simulink model "three_phase_solar_grid"  (R2020b)
settings: Solver=VariableStepAuto  StartTime=0.0  StopTime=0.8  RelTol=1e-6
libraries: powerlib x26, powerlib_meascontrol x3, simulink x3, re_lib x1
settings Model: Creator=a6039  LastModifiedBy=a6039

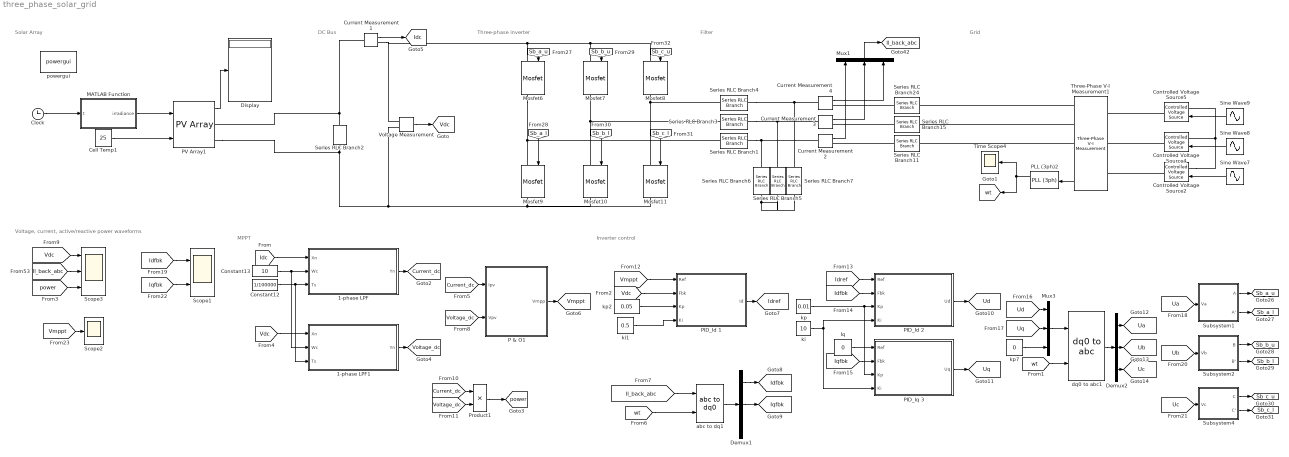
== system three_phase_solar_grid ==
  note: Filter
  note: Solar Array
  note: MPPT
  note: Three-phase inverter
  note: Inverter control
  note: Voltage, current, active/reactive power waveforms
  note: DC Bus
  note: Grid
  1-phase LPF : Subsystem  TreatAsAtomicUnit=on
  1-phase LPF1 : Subsystem  TreatAsAtomicUnit=on
  Cell Temp1 : Constant  Value=25
  Clock : Clock
  Constant12 : Constant  Value=1/100000
  Constant13 : Constant  Value=10
  Controlled Voltage Source2 : powerlib/Electrical Sources/Controlled Voltage Source  Initialize=on  Source_Type=AC  Amplitude=0  Phase=0  Frequency=0  Measurements=None
  Controlled Voltage Source4 : powerlib/Electrical Sources/Controlled Voltage Source  Initialize=on  Source_Type=AC  Amplitude=0  Phase=0  Frequency=0  Measurements=None
  Controlled Voltage Source5 : powerlib/Electrical Sources/Controlled Voltage Source  Initialize=on  Source_Type=AC  Amplitude=0  Phase=0  Frequency=0  Measurements=None
  Current Measurement{1..4} (4 alike) : powerlib/Measurements/Current Measurement  PhasorSimulation=off  OutputType=Complex  PSBequivalent=0
  Demux1 : Demux  Outputs=3
  Demux2 : Demux  Outputs=3
  Display : Display
      settings: Decimation=5
  Iq : Constant  Value=0
  MATLAB Function : MATLAB Function  TreatAsAtomicUnit=on
  Mosfet{6..11} (6 alike) : powerlib/Power Electronics/Mosfet  Ron=0.1  Lon=0  Rd=0.01  Vfd=0  IC=0  Rs=1e5  Cs=inf  Measurements=on
  Mux1 : Mux  Inputs=3
  Mux3 : Mux  Inputs=3
  P & O1 : Subsystem
  PID_Id 1 : Subsystem
  PID_Id 2 : Subsystem
  PID_Iq 3 : Subsystem
  PLL (3ph)2 : powerlib_meascontrol/PLL/PLL (3ph)  Fmin=45  Par_Init=[0, 60]  ParK=[180, 3200, 1]  TcD=1e-4  MaxRateChangeFreq=12  FilterCutOffFreq=25  Ts=0  AGC=on
  PV Array1 : re_lib/Solar/PV Array  Npar=40  Nser=10  PlotType=array @ 1000 W/m2 & specified temperatures  S_vec="[ 1000  800  600 400 200 ]"  Temp_C_vec="[ 45 25  ]"  ModuleName=Ablytek 5MN6C175-A0  PlotWhenSelected=off  Pm=175.0914  Ncell=72  Voc=43.99  Isc=5.17  Vm=36.63  Im=4.78  beta_Voc_pc=-0.3616  alpha_Isc_pc=0.041509  beta_Voc=-0.15907  alpha_Isc=0.002146  IL=5.178  I0=1.7842e-10  nI=0.98852  Rsh=249.6758  Rs=0.38412  RobustModel=off  RobustCellTemperature=313.3991  BAL=off  Tc=1e-6  Tfilter=5e-4
  Product1 : Product
  Scope1 : Scope  NumInputPorts=2
  Scope2 : Scope
  Scope3 : Scope  NumInputPorts=3
  Series RLC Branch1 : powerlib/Elements/Series RLC Branch  LConnTagsString=__new0  RConnTagsString=__new0  BranchType=L  Resistance=1  Inductance=1e-3  SetiL0=off  InitialCurrent=0  Capacitance=1e-3  Setx0=off  InitialVoltage=0  Measurements=None
  Series RLC Branch11 : powerlib/Elements/Series RLC Branch  LConnTagsString=__new0  RConnTagsString=__new0  BranchType=RL  Resistance=0.1  Inductance=1e-9  SetiL0=off  InitialCurrent=0  Capacitance=1e-6  Setx0=off  InitialVoltage=0  Measurements=None
  Series RLC Branch15 : powerlib/Elements/Series RLC Branch  LConnTagsString=__new0  RConnTagsString=__new0  BranchType=RL  Resistance=0.1  Inductance=1e-9  SetiL0=off  InitialCurrent=0  Capacitance=1e-6  Setx0=off  InitialVoltage=0  Measurements=None
  Series RLC Branch2 : powerlib/Elements/Series RLC Branch  LConnTagsString=__new0  RConnTagsString=__new0  BranchType=RC  Resistance=1e-8  Inductance=250e-6  SetiL0=off  InitialCurrent=0  Capacitance=1e-3  Setx0=off  InitialVoltage=300  Measurements=None
  Series RLC Branch24 : powerlib/Elements/Series RLC Branch  LConnTagsString=__new0  RConnTagsString=__new0  BranchType=RL  Resistance=0.1  Inductance=1e-9  SetiL0=off  InitialCurrent=0  Capacitance=1e-6  Setx0=off  InitialVoltage=0  Measurements=None
  Series RLC Branch3 : powerlib/Elements/Series RLC Branch  LConnTagsString=__new0  RConnTagsString=__new0  BranchType=L  Resistance=1  Inductance=1e-3  SetiL0=off  InitialCurrent=0  Capacitance=1e-3  Setx0=off  InitialVoltage=0  Measurements=None
  Series RLC Branch4 : powerlib/Elements/Series RLC Branch  LConnTagsString=__new0  RConnTagsString=__new0  BranchType=L  Resistance=1  Inductance=1e-3  SetiL0=off  InitialCurrent=0  Capacitance=1e-3  Setx0=off  InitialVoltage=0  Measurements=None
  Series RLC Branch5 : powerlib/Elements/Series RLC Branch  LConnTagsString=__new0  RConnTagsString=__new0  BranchType=C  Resistance=1  Inductance=10e-4  SetiL0=off  InitialCurrent=0  Capacitance=1e-4  Setx0=off  InitialVoltage=0  Measurements=None
  Series RLC Branch6 : powerlib/Elements/Series RLC Branch  LConnTagsString=__new0  RConnTagsString=__new0  BranchType=C  Resistance=1  Inductance=10e-4  SetiL0=off  InitialCurrent=0  Capacitance=1e-4  Setx0=off  InitialVoltage=0  Measurements=None
  Series RLC Branch7 : powerlib/Elements/Series RLC Branch  LConnTagsString=__new0  RConnTagsString=__new0  BranchType=C  Resistance=1  Inductance=10e-4  SetiL0=off  InitialCurrent=0  Capacitance=1e-4  Setx0=off  InitialVoltage=0  Measurements=None
  Sine Wave7 : Sin  Amplitude=169.7  Frequency=60*2*pi  SampleTime=0
  Sine Wave8 : Sin  Amplitude=169.7  Frequency=60*2*pi  Phase=-2*pi/3  SampleTime=0
  Sine Wave9 : Sin  Amplitude=169.7  Frequency=60*2*pi  Phase=-4*pi/3  SampleTime=0
  Subsystem1 : Subsystem
  Subsystem2 : Subsystem
  Subsystem4 : Subsystem
  Three-Phase V-I Measurement1 : powerlib/Measurements/Three-Phase V-I Measurement  VoltageMeasurement=phase-to-phase  SetLabelV=off  LabelV=Vabc  Vpu=off  VpuLL=off  CurrentMeasurement=yes  SetLabelI=off  LabelI=Iabc  Ipu=off  Pbase=100e6  Vbase=500e3  OutputType=Complex  PhasorSimulation=off  PSBequivalent=0
  Time Scope4 : Scope
  Voltage Measurement : powerlib/Measurements/Voltage Measurement  PhasorSimulation=off  OutputType=Complex  PSBequivalent=0
  abc to dq1 : powerlib_meascontrol/Transformations/abc to dq0  Alignment=Aligned with phase A axis
  dq0 to abc1 : powerlib_meascontrol/Transformations/dq0 to abc  Alignment=Aligned with phase A axis
  ki : Constant  Value=10
  ki1 : Constant  Value=0.5
  kp : Constant  Value=0.01
  kp2 : Constant  Value=0.05
  kp7 : Constant  Value=0
  powergui : powerlib/powergui  Priority=1  SimulationMode=Discrete  SampleTime=1e-7  frequency=60  Iterations=50  frequencyindice=0  Pbase=100e6  ErrMax=1e-4  UnitsV=kV  UnitsW=MW  buscounter=0  FunctionMessages=off  echomessages=off  EnableUseOfTLC=off  CurrentSourceSwitches=off  DisableSnubberDevices=off  DisableRonSwitches=off  DisableVfSwitches=off  DisplayEquations=off  AutomaticDiscreteSolvers=off  SolverType=Tustin/Backward Euler (TBE)  Interpol=off  ExternalGateDelay=off  methode=off  Ts=100  x0status=blocks  SPID=on  SwTol=0  HookPort=off  NonlinearTolerance=1e-4  nMaxIteration=100  ContinueOnMaxIteration=off  RestoreLinks=warning  ResistiveCurrentMeasurement=off  Frange=[0:2:500]  Ylog=off  Xlog=on  ShowGrid=off  save=off  variable=ZData  structure=current  ZoomFFT=off  StartTime=0.2  cycles=20  DisplayStyle=1  fundamental=50  FreqAxis=off  MaxFrequency=500  frequencyindicesteady=1  RmsSteady=1  display=off
  tag scope: Current_dc=global, Idc=global, Idfbk=global, Idref=global, Il_back_abc=global, Iqfbk=global, Sb_a_l=global, Sb_a_u=global, Sb_b_l=global, Sb_b_u=global, Sb_c_l=global, Sb_c_u=global, Ua=global, Ub=global, Uc=global, Ud=global, Uq=global, Vdc=global, Vmppt=global, Voltage_dc=global, power=global, wt=global
  wires:
  Current Measurement2/1 -> Mux1/1
  Current Measurement3/1 -> Mux1/2
  Current Measurement4/1 -> Mux1/3
  [Il_back_abc] -> Scope3/2
  Iq/1 -> PID_Iq 3/1(Ref)
  abc to dq1/1 -> Demux1/1
  [wt] -> dq0 to abc1/2
  kp/1 -> PID_Iq 3/3(Kp), PID_Id 2/3(Kp)
  ki/1 -> PID_Id 2/4(Ki), PID_Iq 3/4(Ki)
  Mux3/1 -> dq0 to abc1/1
  [wt] -> abc to dq1/2
  dq0 to abc1/1 -> Demux2/1
  PLL (3ph)2/2 -> [wt], Time Scope4/1
  Sine Wave8/1 -> Controlled Voltage Source4/1
  Sine Wave9/1 -> Controlled Voltage Source5/1
  Sine Wave7/1 -> Controlled Voltage Source2/1
  Three-Phase V-I Measurement1/1 -> PLL (3ph)2/1
  [Il_back_abc] -> abc to dq1/1
  Mux1/1 -> [Il_back_abc]
  Cell Temp1/1 -> PV Array1/2
  [Sb_a_u] -> Mosfet6/1
  [Sb_b_u] -> Mosfet7/1
  [Sb_c_u] -> Mosfet8/1
  [Sb_a_l] -> Mosfet9/1
  [Sb_b_l] -> Mosfet10/1
  [Sb_c_l] -> Mosfet11/1
  Voltage Measurement/1 -> [Vdc]
  PV Array1/1 -> Display/1
  [Vdc] -> PID_Id 1/2(Fbk)
  kp2/1 -> PID_Id 1/3(Kp)
  ki1/1 -> PID_Id 1/4(Ki)
  Constant12/1 -> 1-phase LPF1/3(Ts), 1-phase LPF/3(Ts)
  Constant13/1 -> 1-phase LPF1/2(Wc), 1-phase LPF/2(Wc)
  [Idc] -> 1-phase LPF/1(Xn)
  [Vdc] -> 1-phase LPF1/1(Xn)
  Subsystem1/1(A) -> [Sb_a_u]
  Subsystem1/2(A') -> [Sb_a_l]
  Subsystem2/1(B) -> [Sb_b_u]
  Subsystem2/2(B') -> [Sb_b_l]
  Subsystem4/1(C) -> [Sb_c_u]
  Subsystem4/2(C') -> [Sb_c_l]
  kp7/1 -> Mux3/3
  [Vdc] -> Scope3/1
  [power] -> Scope3/3
  Product1/1 -> [power]
  MATLAB Function/1(irradiance) -> PV Array1/1
  Clock/1 -> MATLAB Function/1(t)
  Current Measurement1/1 -> [Idc]
  1-phase LPF/1(Yn) -> [Current_dc]
  1-phase LPF1/1(Yn) -> [Voltage_dc]
  [Current_dc] -> P & O1/1(Ipv)
  [Voltage_dc] -> P & O1/2(Vpv)
  [Current_dc] -> Product1/1
  [Voltage_dc] -> Product1/2
  P & O1/1(Vmpp) -> [Vmppt]
  [Vmppt] -> PID_Id 1/1(Ref)
  PID_Id 1/1(Id) -> [Idref]
  [Idref] -> PID_Id 2/1(Ref)
  Demux1/1 -> [Idfbk]
  Demux1/2 -> [Iqfbk]
  [Idfbk] -> PID_Id 2/2(Fbk)
  [Iqfbk] -> PID_Iq 3/2(Fbk)
  PID_Id 2/1(Ud) -> [Ud]
  PID_Iq 3/1(Uq) -> [Uq]
  [Ud] -> Mux3/1
  [Uq] -> Mux3/2
  Demux2/1 -> [Ua]
  Demux2/2 -> [Ub]
  Demux2/3 -> [Uc]
  [Ua] -> Subsystem1/1(Va)
  [Ub] -> Subsystem2/1(Vb)
  [Uc] -> Subsystem4/1(Vc)
  [Idfbk] -> Scope1/1
  [Iqfbk] -> Scope1/2
  [Vmppt] -> Scope2/1
  connections:
  Mosfet6/LConn1 -- Voltage Measurement/LConn1 -- Current Measurement1/RConn1 -- Mosfet8/LConn1 -- Mosfet7/LConn1
  Mosfet11/LConn1 -- Series RLC Branch4/LConn1 -- Mosfet8/RConn1
  Mosfet10/LConn1 -- Series RLC Branch3/LConn1 -- Mosfet7/RConn1
  Mosfet6/RConn1 -- Mosfet9/LConn1 -- Series RLC Branch1/LConn1
  Controlled Voltage Source2/LConn1 -- Controlled Voltage Source5/LConn1 -- Controlled Voltage Source4/LConn1
  Controlled Voltage Source5/RConn1 -- Three-Phase V-I Measurement1/LConn3
  Controlled Voltage Source2/RConn1 -- Three-Phase V-I Measurement1/LConn1
  Controlled Voltage Source4/RConn1 -- Three-Phase V-I Measurement1/LConn2
  Series RLC Branch2/LConn1 -- PV Array1/RConn2 -- Voltage Measurement/LConn2 -- Mosfet11/RConn1 -- Mosfet10/RConn1 -- Mosfet9/RConn1
  Series RLC Branch6/RConn1 -- Series RLC Branch7/RConn1 -- Series RLC Branch5/RConn1
  Three-Phase V-I Measurement1/RConn1 -- Series RLC Branch11/RConn1
  Three-Phase V-I Measurement1/RConn2 -- Series RLC Branch15/RConn1
  Three-Phase V-I Measurement1/RConn3 -- Series RLC Branch24/RConn1
  Series RLC Branch1/RConn1 -- Series RLC Branch6/LConn1 -- Current Measurement2/LConn1
  Series RLC Branch3/RConn1 -- Series RLC Branch5/LConn1 -- Current Measurement3/LConn1
  Series RLC Branch4/RConn1 -- Series RLC Branch7/LConn1 -- Current Measurement4/LConn1
  Series RLC Branch24/LConn1 -- Current Measurement4/RConn1
  Series RLC Branch15/LConn1 -- Current Measurement3/RConn1
  Series RLC Branch11/LConn1 -- Current Measurement2/RConn1
  Series RLC Branch2/RConn1 -- PV Array1/RConn1 -- Current Measurement1/LConn1

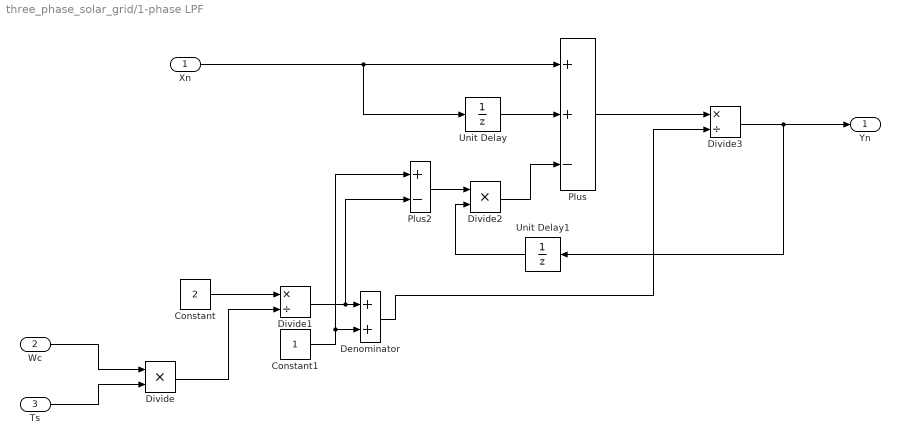
== system three_phase_solar_grid/1-phase LPF ==
  Xn : Inport
  Wc : Inport  Port=2
  Ts : Inport  Port=3
  Constant : Constant  Value=2
  Constant1 : Constant
  Denominator : Sum
  Divide : Product  Inputs=**
  Divide1 : Product  Inputs=*/
  Divide2 : Product  Inputs=**
  Divide3 : Product  Inputs=*/
  Plus : Sum  Inputs=++-
  Plus2 : Sum  Inputs=+-
  Unit Delay : UnitDelay  SampleTime=-1  HasFrameUpgradeWarning=on
  Unit Delay1 : UnitDelay  SampleTime=-1  HasFrameUpgradeWarning=on
  Yn : Outport
  wires:
  Xn/1 -> Unit Delay/1, Plus/1
  Unit Delay/1 -> Plus/2
  Wc/1 -> Divide/1
  Ts/1 -> Divide/2
  Divide/1 -> Divide1/2
  Constant/1 -> Divide1/1
  Divide1/1 -> Plus2/2, Denominator/1
  Constant1/1 -> Plus2/1, Denominator/2
  Plus2/1 -> Divide2/1
  Unit Delay1/1 -> Divide2/2
  Plus/1 -> Divide3/1
  Denominator/1 -> Divide3/2
  Divide3/1 -> Unit Delay1/1, Yn/1
  Divide2/1 -> Plus/3

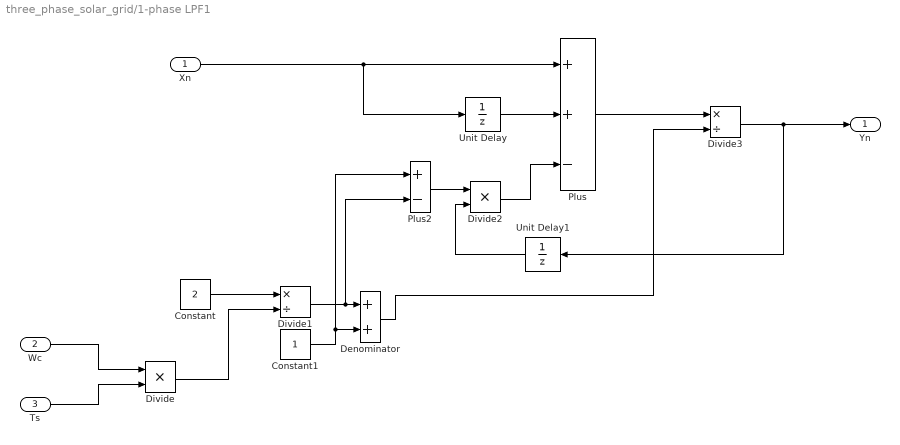
== system three_phase_solar_grid/1-phase LPF1 ==
  Xn : Inport
  Wc : Inport  Port=2
  Ts : Inport  Port=3
  Constant : Constant  Value=2
  Constant1 : Constant
  Denominator : Sum
  Divide : Product  Inputs=**
  Divide1 : Product  Inputs=*/
  Divide2 : Product  Inputs=**
  Divide3 : Product  Inputs=*/
  Plus : Sum  Inputs=++-
  Plus2 : Sum  Inputs=+-
  Unit Delay : UnitDelay  SampleTime=-1  HasFrameUpgradeWarning=on
  Unit Delay1 : UnitDelay  SampleTime=-1  HasFrameUpgradeWarning=on
  Yn : Outport
  wires:
  Xn/1 -> Unit Delay/1, Plus/1
  Unit Delay/1 -> Plus/2
  Wc/1 -> Divide/1
  Ts/1 -> Divide/2
  Divide/1 -> Divide1/2
  Constant/1 -> Divide1/1
  Divide1/1 -> Plus2/2, Denominator/1
  Constant1/1 -> Plus2/1, Denominator/2
  Plus2/1 -> Divide2/1
  Unit Delay1/1 -> Divide2/2
  Plus/1 -> Divide3/1
  Denominator/1 -> Divide3/2
  Divide3/1 -> Unit Delay1/1, Yn/1
  Divide2/1 -> Plus/3

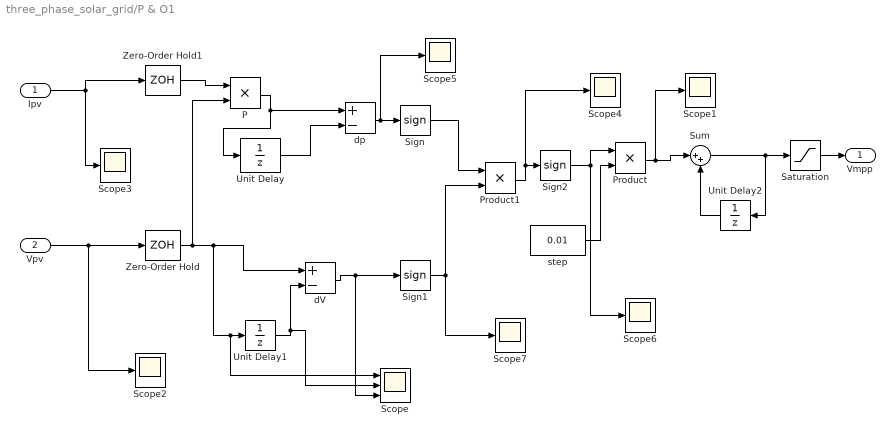
== system three_phase_solar_grid/P & O1 ==
  Ipv : Inport
  Vpv : Inport  Port=2
  P : Product  RndMeth=Zero
  Product : Product  RndMeth=Zero
  Product1 : Product  RndMeth=Zero
  Saturation : Saturate  UpperLimit=450  LowerLimit=0  LinearizeAsGain=off  ZeroCross=off
  Scope : Scope  NumInputPorts=3
  Scope{1..7} (7 alike) : Scope
  Sign : Signum
  Sign1 : Signum
  Sign2 : Signum
  Sum : Sum  Inputs=|++
  Unit Delay : UnitDelay  SampleTime=-1  HasFrameUpgradeWarning=on
  Unit Delay1 : UnitDelay  SampleTime=-1  HasFrameUpgradeWarning=on
  Unit Delay2 : UnitDelay  InitialCondition=400  SampleTime=-1  HasFrameUpgradeWarning=on
  Zero-Order Hold : ZeroOrderHold  SampleTime=1/100000
  Zero-Order Hold1 : ZeroOrderHold  SampleTime=1/100000
  dV : Sum  Inputs=+-
  dp : Sum  Inputs=+-
  step : Constant  Value=0.01
  Vmpp : Outport
  wires:
  Unit Delay1/1 -> dV/2, Scope/2
  Unit Delay/1 -> dp/2
  dV/1 -> Sign1/1, Scope/3
  step/1 -> Product/2
  Product/1 -> Sum/1, Scope1/1
  Sign/1 -> Product1/1
  Sign1/1 -> Product1/2, Scope7/1
  Product1/1 -> Sign2/1, Scope4/1
  Ipv/1 -> Scope3/1, Zero-Order Hold1/1
  Vpv/1 -> Zero-Order Hold/1, Scope2/1
  P/1 -> Unit Delay/1, dp/1
  dp/1 -> Sign/1, Scope5/1
  Sign2/1 -> Product/1, Scope6/1
  Sum/1 -> Saturation/1, Unit Delay2/1
  Unit Delay2/1 -> Sum/2
  Zero-Order Hold/1 -> P/2, Scope/1, Unit Delay1/1, dV/1
  Zero-Order Hold1/1 -> P/1
  Saturation/1 -> Vmpp/1

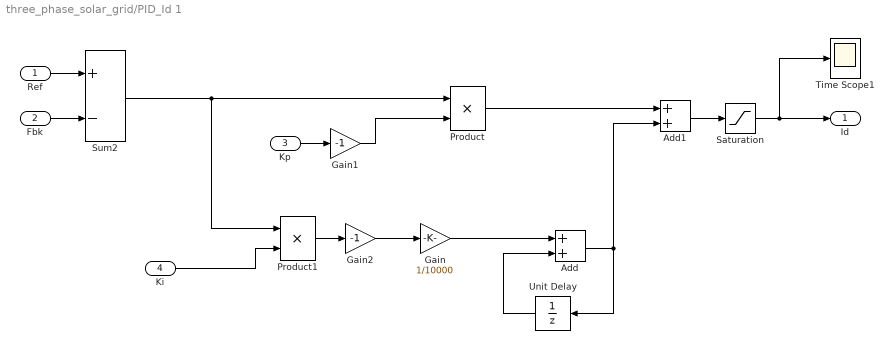
== system three_phase_solar_grid/PID_Id 1 ==
  Ref : Inport
  Fbk : Inport  Port=2
  Kp : Inport  Port=3
  Ki : Inport  Port=4
  Add : Sum
  Add1 : Sum
  Gain : Gain  Gain=1/10000
  Gain1 : Gain  Gain=-1
  Gain2 : Gain  Gain=-1
  Product : Product  OutDataTypeStr=Inherit: Same as first input
  Product1 : Product  OutDataTypeStr=Inherit: Same as first input
  Saturation : Saturate  UpperLimit=1000  LowerLimit=0  LinearizeAsGain=off  ZeroCross=off
  Sum2 : Sum  Inputs=+-
  Time Scope1 : Scope
  Unit Delay : UnitDelay  SampleTime=-1  HasFrameUpgradeWarning=on
  Id : Outport
  wires:
  Sum2/1 -> Product1/1, Product/1
  Fbk/1 -> Sum2/2
  Ref/1 -> Sum2/1
  Product1/1 -> Gain2/1
  Add/1 -> Unit Delay/1, Add1/2
  Product/1 -> Add1/1
  Gain/1 -> Add/1
  Unit Delay/1 -> Add/2
  Kp/1 -> Gain1/1
  Ki/1 -> Product1/2
  Gain1/1 -> Product/2
  Gain2/1 -> Gain/1
  Add1/1 -> Saturation/1
  Saturation/1 -> Time Scope1/1, Id/1

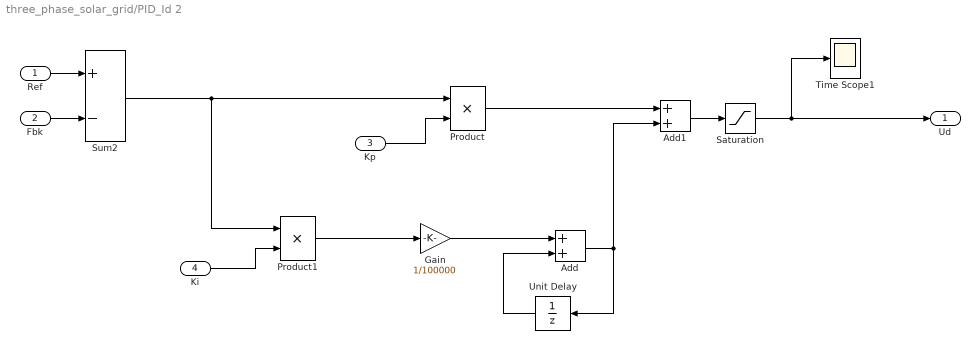
== system three_phase_solar_grid/PID_Id 2 ==
  Ref : Inport
  Fbk : Inport  Port=2
  Kp : Inport  Port=3
  Ki : Inport  Port=4
  Add : Sum
  Add1 : Sum
  Gain : Gain  Gain=1/100000
  Product : Product  OutDataTypeStr=Inherit: Same as first input
  Product1 : Product  OutDataTypeStr=Inherit: Same as first input
  Saturation : Saturate  UpperLimit=500  LowerLimit=-500  LinearizeAsGain=off  ZeroCross=off
  Sum2 : Sum  Inputs=+-
  Time Scope1 : Scope
  Unit Delay : UnitDelay  InitialCondition=400  SampleTime=-1  HasFrameUpgradeWarning=on
  Ud : Outport
  wires:
  Add1/1 -> Saturation/1
  Sum2/1 -> Product1/1, Product/1
  Fbk/1 -> Sum2/2
  Ref/1 -> Sum2/1
  Kp/1 -> Product/2
  Ki/1 -> Product1/2
  Product1/1 -> Gain/1
  Add/1 -> Unit Delay/1, Add1/2
  Product/1 -> Add1/1
  Saturation/1 -> Time Scope1/1, Ud/1
  Gain/1 -> Add/1
  Unit Delay/1 -> Add/2

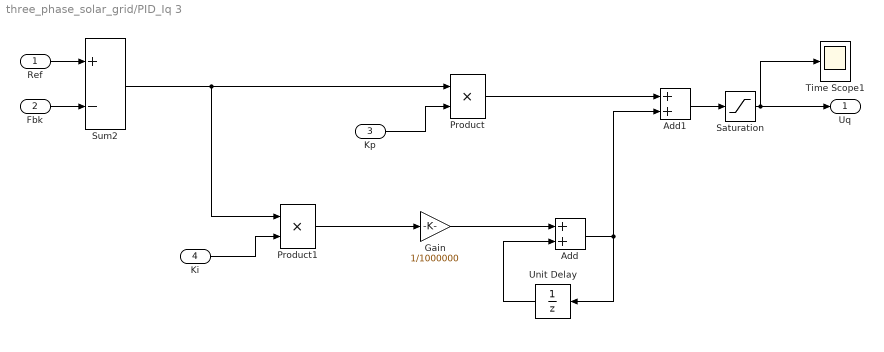
== system three_phase_solar_grid/PID_Iq 3 ==
  Ref : Inport
  Fbk : Inport  Port=2
  Kp : Inport  Port=3
  Ki : Inport  Port=4
  Add : Sum
  Add1 : Sum
  Gain : Gain  Gain=1/1000000
  Product : Product  OutDataTypeStr=Inherit: Same as first input
  Product1 : Product  OutDataTypeStr=Inherit: Same as first input
  Saturation : Saturate  UpperLimit=500  LowerLimit=-500  LinearizeAsGain=off  ZeroCross=off
  Sum2 : Sum  Inputs=+-
  Time Scope1 : Scope
  Unit Delay : UnitDelay  SampleTime=-1  HasFrameUpgradeWarning=on
  Uq : Outport
  wires:
  Add1/1 -> Saturation/1
  Sum2/1 -> Product1/1, Product/1
  Fbk/1 -> Sum2/2
  Ref/1 -> Sum2/1
  Kp/1 -> Product/2
  Ki/1 -> Product1/2
  Product1/1 -> Gain/1
  Add/1 -> Unit Delay/1, Add1/2
  Product/1 -> Add1/1
  Gain/1 -> Add/1
  Unit Delay/1 -> Add/2
  Saturation/1 -> Time Scope1/1, Uq/1

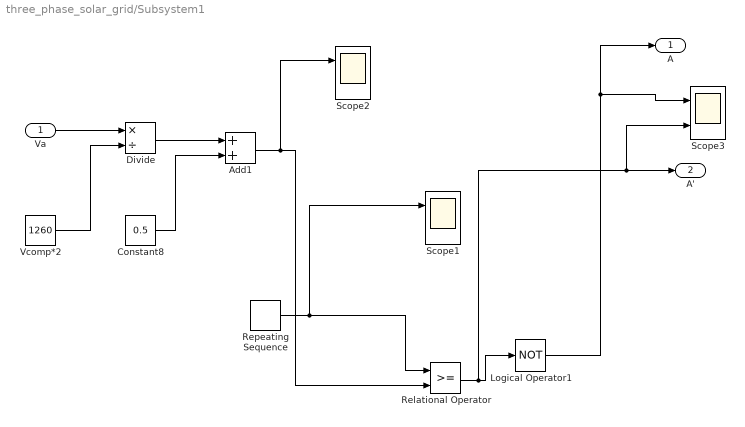
== system three_phase_solar_grid/Subsystem1 ==
  Va : Inport
  Add1 : Sum
  Constant8 : Constant  Value=0.5
  Divide : Product  Inputs=*/
  Logical Operator1 : Logic  Operator=NOT  AllPortsSameDT=off  OutDataTypeStr=boolean
  Relational Operator : RelationalOperator  OutDataTypeStr=boolean  ZeroCross=off  RndMeth=Nearest
  Repeating Sequence : simulink/Sources/Repeating Sequence  rep_seq_t=[0 1/100000/2 1/100000]  rep_seq_y=[0 1 0]
  Scope1 : Scope  NumInputPorts=2
  Scope2 : Scope  NumInputPorts=2
  Scope3 : Scope  NumInputPorts=2
  Vcomp*2 : Constant  Value=1260
  A : Outport
  A' : Outport  Port=2
  wires:
  Va/1 -> Divide/1
  Divide/1 -> Add1/1
  Add1/1 -> Scope2/1, Relational Operator/2
  Constant8/1 -> Add1/2
  Repeating Sequence/1 -> Scope1/1, Relational Operator/1
  Logical Operator1/1 -> Scope3/1, A/1
  Relational Operator/1 -> Scope3/2, A'/1, Logical Operator1/1
  Vcomp*2/1 -> Divide/2

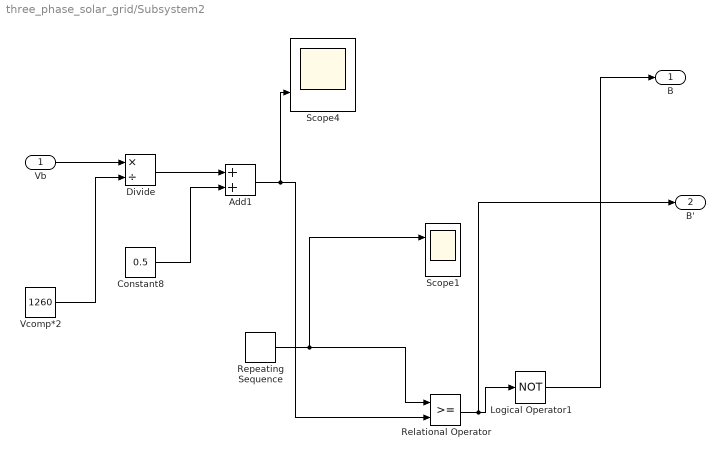
== system three_phase_solar_grid/Subsystem2 ==
  Vb : Inport
  Add1 : Sum
  Constant8 : Constant  Value=0.5
  Divide : Product  Inputs=*/
  Logical Operator1 : Logic  Operator=NOT  AllPortsSameDT=off  OutDataTypeStr=boolean
  Relational Operator : RelationalOperator  OutDataTypeStr=boolean  ZeroCross=off  RndMeth=Nearest
  Repeating Sequence : simulink/Sources/Repeating Sequence  rep_seq_t=[0 1/100000/2 1/100000]  rep_seq_y=[0 1 0]
  Scope1 : Scope  NumInputPorts=2
  Scope4 : Scope  NumInputPorts=2
  Vcomp*2 : Constant  Value=1260
  B : Outport
  B' : Outport  Port=2
  wires:
  Vb/1 -> Divide/1
  Divide/1 -> Add1/1
  Add1/1 -> Relational Operator/2, Scope4/2
  Constant8/1 -> Add1/2
  Repeating Sequence/1 -> Scope1/1, Relational Operator/1
  Logical Operator1/1 -> B/1
  Relational Operator/1 -> B'/1, Logical Operator1/1
  Vcomp*2/1 -> Divide/2

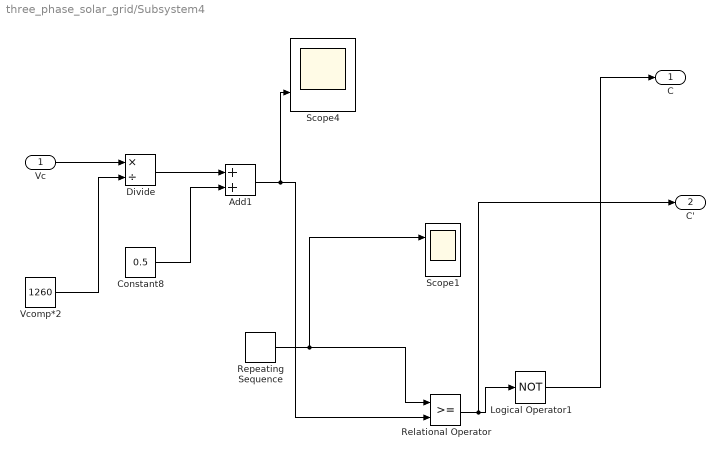
== system three_phase_solar_grid/Subsystem4 ==
  Vc : Inport
  Add1 : Sum
  Constant8 : Constant  Value=0.5
  Divide : Product  Inputs=*/
  Logical Operator1 : Logic  Operator=NOT  AllPortsSameDT=off  OutDataTypeStr=boolean
  Relational Operator : RelationalOperator  OutDataTypeStr=boolean  ZeroCross=off  RndMeth=Nearest
  Repeating Sequence : simulink/Sources/Repeating Sequence  rep_seq_t=[0 1/100000/2 1/100000]  rep_seq_y=[0 1 0]
  Scope1 : Scope  NumInputPorts=2
  Scope4 : Scope  NumInputPorts=2
  Vcomp*2 : Constant  Value=1260
  C : Outport
  C' : Outport  Port=2
  wires:
  Vc/1 -> Divide/1
  Divide/1 -> Add1/1
  Add1/1 -> Relational Operator/2, Scope4/2
  Constant8/1 -> Add1/2
  Repeating Sequence/1 -> Scope1/1, Relational Operator/1
  Logical Operator1/1 -> C/1
  Relational Operator/1 -> C'/1, Logical Operator1/1
  Vcomp*2/1 -> Divide/2

== matlab function three_phase_solar_grid/MATLAB Function ==
  data: irradiance output; t input
function irradiance     =   init(t)

if t<0.3
    irradiance=1000;
    
elseif t<0.5
    irradiance=800;
    
else
   irradiance=1000;

end
